simulink subsystem "blood_joint"  (R2020b)
settings: Solver=VariableStepAuto  StartTime=0.0  StopTime=10.0  RelTol=1e-3
settings Model: Creator=RH  LastModifiedBy=Marco

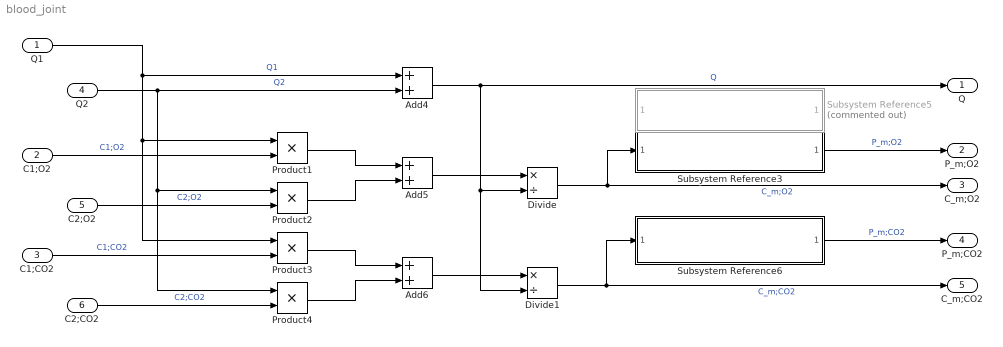
== system blood_joint ==
  Q1 : Inport  Unit=liter/minute
  C1;O2 : Inport  Port=2  Unit=1
  C1;CO2 : Inport  Port=3  Unit=1
  Q2 : Inport  Port=4  Unit=liter/minute
  C2;O2 : Inport  Port=5  Unit=1
  C2;CO2 : Inport  Port=6  Unit=1
  Add4 : Sum
  Add5 : Sum
  Add6 : Sum
  Divide : Product  Inputs=*/
  Divide1 : Product  Inputs=*/
  Product{1..4} (4 alike) : Product
  Subsystem Reference3 : Subsystem  ReferencedSubsystem=O2_dissociation_inv
  Subsystem Reference5 : Subsystem  Commented=on  ReferencedSubsystem=O2_dissociation_inv_poly
  Subsystem Reference6 : Subsystem  ReferencedSubsystem=CO2_dissociation_inv
  Q : Outport  Unit=liter/minute
  P_m;O2 : Outport  Port=2  Unit=mmHg
  C_m;O2 : Outport  Port=3  Unit=1
  P_m;CO2 : Outport  Port=4  Unit=mmHg
  C_m;CO2 : Outport  Port=5  Unit=1
  wires:
  Add4/1 -> Divide1/2, Divide/2, Q/1  "Q"
  Product1/1 -> Add5/1
  C1;O2/1 -> Product1/2  "C1;O2"
  Divide1/1 -> Subsystem Reference6/1, C_m;CO2/1  "C_m;CO2"
  Q2/1 -> Add4/2, Product2/1, Product4/1  "Q2"
  C1;CO2/1 -> Product3/2  "C1;CO2"
  Q1/1 -> Add4/1, Product3/1, Product1/1  "Q1"
  Divide/1 -> Subsystem Reference3/1, C_m;O2/1  "C_m;O2"
  Subsystem Reference3/1 -> P_m;O2/1  "P_m;O2"
  Add5/1 -> Divide/1
  Add6/1 -> Divide1/1
  Product2/1 -> Add5/2
  Product3/1 -> Add6/1
  Subsystem Reference6/1 -> P_m;CO2/1  "P_m;CO2"
  Product4/1 -> Add6/2
  C2;O2/1 -> Product2/2  "C2;O2"
  C2;CO2/1 -> Product4/2  "C2;CO2"
